simulink model "simulink_kalman"  (R2025b)
settings: Solver=ode4  StartTime=0.0  StopTime=30  FixedStep=0.001  RelTol=1e-3
values from neighbouring files (symbols this model uses):
  A = 20    [sinus_transport.m]    (also in state_models.m = sys_d.A)
  B = sys_d.B    [state_models.m]
  C = Kp*(1 + 1/(Ti*s))    [simc_tuning.m]    (also in state_models.m = sys_d.C)
  K = params(1)    [simc_tuning.m]
  Kp = 7.43060221924    [pid_params.mat]    (also in simc_tuning.m = T / (K * (tau_c + t0)))
  Q = eye(2) * best_result(1)    [R_Q_script.m]
  R = best_result(2)    [R_Q_script.m]
  T = params(2)/6500    [simc_tuning.m]
  Ti = 0.0100898358758    [pid_params.mat]    (also in simc_tuning.m = min(T, 4*(tau_c + t0)))
libraries: slpidlib x1
settings Model: Creator=00ary  LastModifiedBy=00ary
settings DebuggingCC: AlgebraicLoopMsg=none

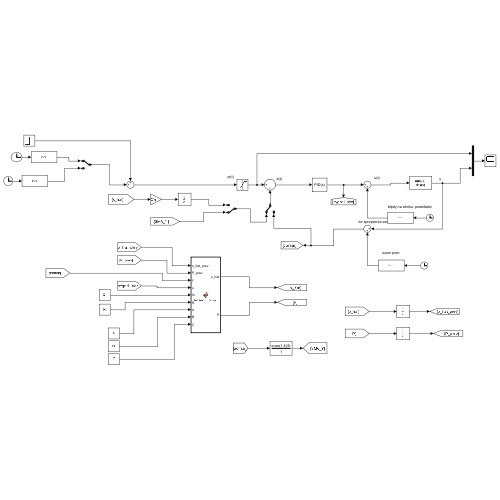
[thumbnail: Simulink's stored preview of the top-level diagram]
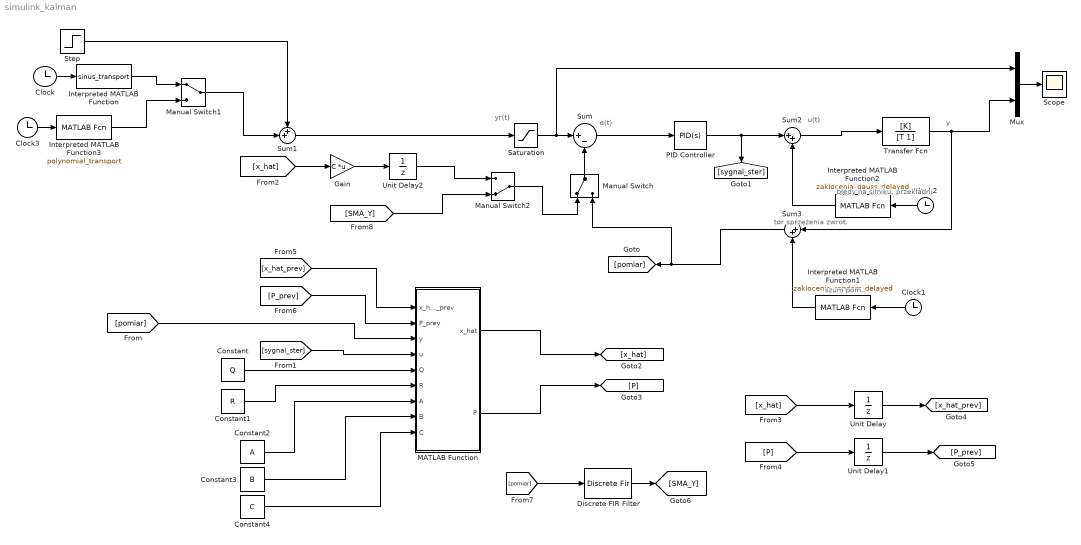
== system simulink_kalman ==
  note: u(t)
  note: tor sprzężenia zwrot.
  note: y
  note: błędy na silniku, przekładni
  note: szum pom.
  note: e(t)
  note: yr(t)
  Clock{,1..3} (4 alike) : Clock
      Clock settings: Decimation=100
      Clock3 settings: Decimation=100
  Constant : Constant  Value=Q
  Constant1 : Constant  Value=R
  Constant2 : Constant  Value=A
  Constant3 : Constant  Value=B
  Constant4 : Constant  Value=C
  Discrete FIR Filter : DiscreteFir  Coefficients=[ones(1,8)/8]
  Gain : Gain  Gain=C  Multiplication=Matrix(K*u)
  Interpreted MATLAB Function : MATLABFcn  MATLABFcn=sinus_transport
  Interpreted MATLAB Function1 : MATLABFcn  MATLABFcn=zaklocenia_random_delayed
  Interpreted MATLAB Function2 : MATLABFcn  MATLABFcn=zaklocenia_gauss_delayed
  Interpreted MATLAB Function3 : MATLABFcn  MATLABFcn=polynomial_transport
  MATLAB Function : MATLAB Function  TreatAsAtomicUnit=on
  Manual Switch : ManualSwitch
  Manual Switch1 : ManualSwitch
  Manual Switch2 : ManualSwitch  CurrentSetting=0
  Mux : Mux  Inputs=2
  PID Controller : slpidlib/PID Controller  Controller=PID  Form=Ideal  TimeDomain=Continuous-time  UseExternalTs=off  SampleTime=-1  IntegratorMethod=Forward Euler  FilterMethod=Forward Euler  ControllerParametersSource=internal  P=Kp  I=Ti*1000  UseKiTs=off  D=0  UseExternalDerivativeSource=off  N=100  UseFilter=on  TunerSelectOption=Transfer Function Based (PID Tuner App)  InitialConditionSource=internal  InitialConditionForIntegrator=0  InitialConditionForFilter=0  DifferentiatorICPrevScaledInput=0  ExternalReset=none  TrackingMode=off  Kt=1  LimitOutput=off  SatLimitsSource=internal  UpperSaturationLimit=inf  LowerSaturationLimit=-inf  LinearizeAsGain=on  AntiWindupMode=none  Kb=1  LimitIntegrator=off  UpperIntegratorSaturationLimit=inf  LowerIntegratorSaturationLimit=-inf  POutMin=[]  POutMax=[]  IOutMin=[]  IOutMax=[]  DOutMin=[]  DOutMax=[]  NOutMin=[]  NOutMax=[]  SumOutMin=[]  SumOutMax=[]  SaturationOutMin=[]  SaturationOutMax=[]  PParamMin=[]  PParamMax=[]  IParamMin=[]  IParamMax=[]  DParamMin=[]  DParamMax=[]  NParamMin=[]  NParamMax=[]  KbParamMin=[]  KbParamMax=[]  KtParamMin=[]  KtParamMax=[]  KbOutMin=[]  KbOutMax=[]  KtOutMin=[]  KtOutMax=[]  IntegratorOutMin=[]  IntegratorOutMax=[]  FilterOutMin=[]  FilterOutMax=[]  SumI1OutMin=[]  SumI1OutMax=[]  SumI2OutMin=[]  SumI2OutMax=[]  SumI3OutMin=[]  SumI3OutMax=[]  SumI4OutMin=[]  SumI4OutMax=[]  SumDOutMin=[]  SumDOutMax=[]  DifferentiatorOutMin=[]  DifferentiatorOutMax=[]  FilterDiffOutCoefMin=[]  FilterDiffOutCoefMax=[]  ReciprocalOutMin=[]  ReciprocalOutMax=[]  SumDenOutMin=[]  SumDenOutMax=[]  SumNumOutMin=[]  SumNumOutMax=[]  DivideOutMin=[]  DivideOutMax=[]  UdiffTsProdOutMin=[]  UdiffTsProdOutMax=[]  NTsProdOutMin=[]  NTsProdOutMax=[]  UintegralTsProdOutMin=[]  UintegralTsProdOutMax=[]  UngainTsProdOutMin=[]  UngainTsProdOutMax=[]  ClampingZeroOutDataTypeStr=Inherit: Inherit via back propagation  ClampingZeroOutMin=[]  ClampingZeroOutMax=[]  FilterDenConstantOutDataTypeStr=Inherit: Inherit via back propagation  FilterDenConstantOutMin=[]  FilterDenConstantOutMax=[]  PCopyOutDataTypeStr=Inherit: Inherit via back propagation  PCopyOutMin=[]  PCopyOutMax=[]  NCopyOutDataTypeStr=Inherit: Inherit via back propagation  NCopyOutMin=[]  NCopyOutMax=[]  IntegratorContinuousStateAttributes=''  IntegratorStateMustResolveToSignalObject=off  IntegratorRTWStateStorageClass=Auto  FilterContinuousStateAttributes=''  FilterStateMustResolveToSignalObject=off  FilterRTWStateStorageClass=Auto  ParallelPVariant=Passthrough  IdealPVariant=InternalParameters  IVariant=InternalParameters  DVariant=InternalParameters  IntegratorVariant=Continuous  SatVariant=Disabled  AWVariant=Passthrough  PCopyVariant=Disabled  TRVariant=Disabled  FdbkBlocksVariant=Forward  IdealPFdbkVariant=Disabled  SatFdbkVariant=Disabled  DerivativeFilterVariant=ContFilter  NVariant=InternalParameters  NCopyVariant=Disabled  FilterICVariant=InternalICsFilter  IntegratorICVariant=InternalICs  ExternalResetVariant=Disabled  TRSumVariant=Passthrough  SumFdbkVariant=Disabled  SumVariant=Sum_PID  TsampFilterVariant=InternalTs  TsampNgainVariant=Passthrough  TsampIntegralVariant=Disabled_SignalSpec  ExternalSaturationOutDataTypeStr=Inherit: Same as second input  DerivativeSourceVariant=ErrorSignal  PreIntVariant=InternalPreInt
  Saturation : Saturate  UpperLimit=250  LowerLimit=0
  Scope : Scope
      settings: ActiveDisplayYMinimum=51.154067014555928  ActiveDisplayYMaximum=65.906616299895546
  Step : Step  After=40  SampleTime=0
  Sum : Sum  Inputs=|+-
  Sum1 : Sum  Inputs=++|
  Sum2 : Sum  Inputs=|++
  Sum3 : Sum  Inputs=|++
  Transfer Fcn : TransferFcn  Numerator=[K]  Denominator=[T 1]
  Unit Delay : UnitDelay  SampleTime=-1  HasFrameUpgradeWarning=on
  Unit Delay1 : UnitDelay  SampleTime=-1  HasFrameUpgradeWarning=on
  Unit Delay2 : UnitDelay  SampleTime=-1  HasFrameUpgradeWarning=on
  wires:
  Mux/1 -> Scope/1
  Clock1/1 -> Interpreted MATLAB Function1/1
  Interpreted MATLAB Function2/1 -> Sum2/2
  Transfer Fcn/1 -> Mux/2, Sum3/1
  Interpreted MATLAB Function1/1 -> Sum3/2
  [x_hat_prev] -> MATLAB Function/1(x_hat_prev)
  [pomiar] -> MATLAB Function/3(y)
  [sygnal_ster] -> MATLAB Function/4(u)
  MATLAB Function/1(x_hat) -> [x_hat]
  [P] -> Unit Delay1/1
  [x_hat] -> Unit Delay/1
  Unit Delay/1 -> [x_hat_prev]
  Unit Delay1/1 -> [P_prev]
  Constant/1 -> MATLAB Function/5(Q)
  Constant1/1 -> MATLAB Function/6(R)
  [P_prev] -> MATLAB Function/2(P_prev)
  MATLAB Function/2(P) -> [P]
  Constant2/1 -> MATLAB Function/7(A)
  Constant3/1 -> MATLAB Function/8(B)
  Constant4/1 -> MATLAB Function/9(C)
  Sum3/1 -> Manual Switch/2, [pomiar]
  Step/1 -> Sum1/1
  PID Controller/1 -> Sum2/1, [sygnal_ster]
  [x_hat] -> Gain/1
  Gain/1 -> Unit Delay2/1
  Clock/1 -> Interpreted MATLAB Function/1
  Clock3/1 -> Interpreted MATLAB Function3/1
  Clock2/1 -> Interpreted MATLAB Function2/1
  Sum2/1 -> Transfer Fcn/1
  Sum/1 -> PID Controller/1
  Saturation/1 -> Mux/1, Sum/1
  Sum1/1 -> Saturation/1
  Manual Switch/1 -> Sum/2
  Interpreted MATLAB Function/1 -> Manual Switch1/1
  Interpreted MATLAB Function3/1 -> Manual Switch1/2
  Manual Switch1/1 -> Sum1/2
  Manual Switch2/1 -> Manual Switch/1
  Unit Delay2/1 -> Manual Switch2/1
  [SMA_Y] -> Manual Switch2/2
  [pomiar] -> Discrete FIR Filter/1
  Discrete FIR Filter/1 -> [SMA_Y]

== matlab function simulink_kalman/MATLAB Function ==
  data: x_hat_prev input; P_prev input; y input; u input size=[1 1]; x_hat output; Q input; R input; P output; A input; B input; C input
function [x_hat, P] = kalman_step(x_hat_prev, P_prev, y, u, Q, R, A, B, C)

C = C(:)';

x_pred = A*x_hat_prev + B*u;

P_pred = A*P_prev*A' + Q;

K_kalman = P_pred * C' / (C * P_pred * C' + R);
x_hat = x_pred + K_kalman * (y - C * x_pred);
P = (eye(2) - K_kalman * C) * P_pred;



end
